simulink model "TorqueVectoring"  (R2020b)
settings: Solver=FixedStepAuto  StartTime=0.0  StopTime=Ts  FixedStep=0.001  RelTol=1e-3
PreLoadFcn:
  | setUpPurePursuitCurveHighVel
model workspace (MAT data in the model file):
  firstWarning = 0
  originalScenarioChecksum = 'F73A6DA3C723D3CA73A6F931B7A52A9C'
values from neighbouring files (symbols this model uses):
  Cf = 34282    [matlab.mat]    (also in matlab2.mat)
  Cr = 34282    [matlab.mat]    (also in matlab2.mat)
  g = 9.81    [matlab.mat]    (also in matlab2.mat)
  i = 5.45    [matlab.mat]    (also in matlab2.mat)
  Iz = 162    [matlab.mat]    (also in matlab2.mat)
  lf = 0.686    [matlab.mat]    (also in matlab2.mat)
  lr = 0.838    [matlab.mat]    (also in matlab2.mat)
  m = 300    [matlab.mat]    (also in matlab2.mat)
  period = 0.01    [matlab2.mat]
  Rw = 0.265    [matlab.mat]    (also in matlab2.mat)
  sigma = 1    [matlab.mat]    (also in matlab2.mat)
  tr = 0.549    [matlab.mat]    (also in matlab2.mat)
undefined symbols (not defined in the file or in its folder): Kd, Ki, Kp, MMax
libraries: simulink x2, vehdynlibsteering x1, pid_lib x1
settings Model: EnablePacing=on  PacingRate=0.450000  Creator=valakshe  LastModifiedBy=lugh8
settings SolverCC: ZeroCrossAlgorithm=Adaptive  PositivePriorityOrder=on
settings DataIOCC: SaveOutput=off  SaveTime=off
settings OptimizationCC: DefaultParameterBehavior=Inlined  UseDivisionForNetSlopeComputation=on  GainParamInheritBuiltInType=on  UseFloatMulNetSlope=on  InlineInvariantSignals=on  PassReuseOutputArgsAs=Individual arguments  ZeroExternalMemoryAtStartup=off  ZeroInternalMemoryAtStartup=off  NoFixptDivByZeroProtection=on  EfficientFloat2IntCast=on  LifeSpan=1  MaxStackSize=64  OptimizeBlockOrder=speed  DifferentSizesBufferReuse=on  EfficientTunableParamExpr=on
settings DebuggingCC: IgnoredZcDiagnostic=none  ParameterTunabilityLossMsg=error
settings HardwareCC: ProdBitPerPointer=32  ProdBitPerSizeT=32  ProdBitPerPtrDiffT=32  ProdLargestAtomicInteger=Long  ProdLargestAtomicFloat=Double  ProdWordSize=32  ProdLongLongMode=on  ProdHWDeviceType=ARM Compatible->ARM Cortex-M  HardwareBoardFeatureSet=SoCBlockset
settings SFSimCC: MATLABDynamicMemAlloc=off
settings RTWCC: Description=Embedded Coder  SystemTargetFile=ert.tlc  GenCodeOnly=on  PackageGeneratedCodeAndArtifacts=on  TemplateMakefile=ert_default_tmf
settings CodeAppCC: ForceParamTrailComments=on  IgnoreCustomStorageClasses=off  OperatorAnnotations=on  SimulinkDataObjDesc=on  SFDataObjDesc=on  CustomSymbolStrGlobalVar=rt$N$M  CustomSymbolStrType=$N$M  CustomSymbolStrFcn=$N$M$F  CustomSymbolStrMacro=$N$M  InsertBlockDesc=on
settings ERTTargetCC: IncludeMdlTerminateFcn=off  CombineSignalStateStructs=on  SupportAbsoluteTime=off  SupportComplex=off  SupportContinuousTime=on  SupportNonInlinedSFcns=on  InlinedParameterPlacement=NonHierarchical  ERTCustomFileTemplate=example_file_process.tlc  ERTFilePackagingFormat=CompactWithDataFile

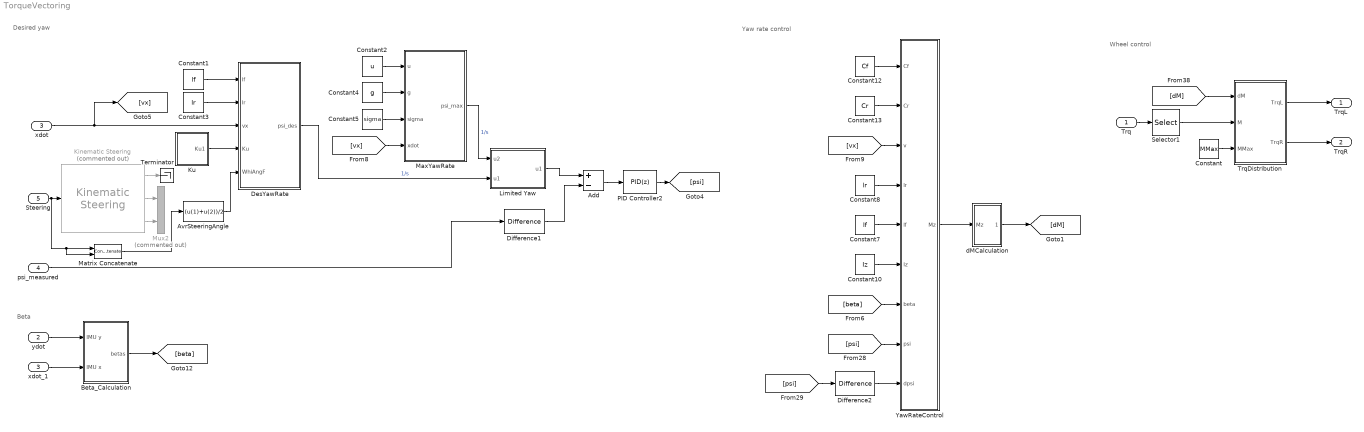
== system TorqueVectoring ==
  note: Desired yaw
  note: Beta
  note: Yaw rate control
  note: Wheel control
  Trq : Inport  OutDataTypeStr=double  PortDimensions=4  SampleTime=0
  ydot : Inport  Port=2  OutDataTypeStr=double  PortDimensions=1  SampleTime=0
  xdot : Inport  Port=3  OutDataTypeStr=double  PortDimensions=1  SampleTime=0
  psi_measured : Inport  Port=4  OutDataTypeStr=double  PortDimensions=1
  Steering : Inport  Port=5  OutDataTypeStr=double  PortDimensions=[1 1]  SampleTime=0
  Add : Sum  Inputs=+-
  AvrSteeringAngle : Fcn  Expr=(u(1)+u(2))/2
  Beta_Calculation : Subsystem
  Constant : Constant  Value=MMax
  Constant1 : Constant  Value=lf
  Constant10 : Constant  Value=Iz
  Constant12 : Constant  Value=Cf
  Constant13 : Constant  Value=Cr
  Constant2 : Constant  Value=u
  Constant3 : Constant  Value=lr
  Constant4 : Constant  Value=g
  Constant5 : Constant  Value=sigma
  Constant7 : Constant  Value=lf
  Constant8 : Constant  Value=lr
  DesYawRate : MATLAB Function  TreatAsAtomicUnit=on
  Difference1 : simulink/Discrete/Difference  ICPrevInput=0.0  OutMin=[]  OutMax=[]  OutDataType=fixdt(1, 16)  OutScaling=2^-10  DoSatur=off
  Difference2 : simulink/Discrete/Difference  ICPrevInput=0.0  OutMin=[]  OutMax=[]  OutDataType=fixdt(1, 16)  OutScaling=2^-10  DoSatur=off
  Kinematic Steering : vehdynlibsteering/Kinematic Steering  Commented=on  StrgType=Ackerman  StrgRatioType=Constant  Loc=Front  NrmlFctr=0.01  TrckWdth=1.098  WhlBase=L  Db=0  StrgRng=3.665  StrgAngBpts="[-6.2832   -5.0265   -3.7699   -2.5133   -1.2566         0    1.2566    2.5133    3.7699    5.0265    6.2832]"  StrgRatioTbl=|  StrgRatio=SR  StrgArmLngth=0.08  RckCsLngth=0.29  TieRodLngth=0.458  D=0.03  PnnRadius=0.019  PnnRadiusTbl="[0.0055    0.0055    0.0056    0.0057    0.0058    0.0057    0.0057    0.0057    0.0056    0.0055    0.0055]"  RodLngth=0.1  ParaArmLngth=0.9  aMode=2
      | [13.5000   13.3750   13.2500   13.1250   13.0000   13.0000   13.0000   13.1250   13.2500   13.3750   13.5000
      | ]
  Ku : Subsystem
  Limited Yaw : MATLAB Function  TreatAsAtomicUnit=on
  Matrix Concatenate : Concatenate
  MaxYawRate : MATLAB Function  TreatAsAtomicUnit=on
  Mux2 : Mux  Commented=on  Inputs=2
  PID Controller2 : pid_lib/PID Controller  Controller=PID  Form=Parallel  TimeDomain=Discrete-time  UseExternalTs=off  SampleTime=period  IntegratorMethod=Forward Euler  FilterMethod=Forward Euler  ControllerParametersSource=internal  P=Kp  I=Ki  D=Kd  UseFilter=on  N=10  TunerSelectOption=Transfer Function Based (PID Tuner App)  InitialConditionSource=internal  InitialConditionForIntegrator=0  InitialConditionForFilter=0  DifferentiatorICPrevScaledInput=0  ExternalReset=none  TrackingMode=off  Kt=1  LimitOutput=on  SatLimitsSource=internal  UpperSaturationLimit=inf  LowerSaturationLimit=-inf  LinearizeAsGain=on  AntiWindupMode=clamping  Kb=1  POutMin=[]  POutMax=[]  IOutMin=[]  IOutMax=[]  DOutMin=[]  DOutMax=[]  NOutMin=[]  NOutMax=[]  SumOutMin=[]  SumOutMax=[]  SaturationOutMin=[]  SaturationOutMax=[]  PParamMin=[]  PParamMax=[]  IParamMin=[]  IParamMax=[]  DParamMin=[]  DParamMax=[]  NParamMin=[]  NParamMax=[]  KbParamMin=[]  KbParamMax=[]  KtParamMin=[]  KtParamMax=[]  KbOutMin=[]  KbOutMax=[]  KtOutMin=[]  KtOutMax=[]  IntegratorOutMin=[]  IntegratorOutMax=[]  FilterOutMin=[]  FilterOutMax=[]  SumI1OutMin=[]  SumI1OutMax=[]  SumI2OutMin=[]  SumI2OutMax=[]  SumI3OutMin=[]  SumI3OutMax=[]  SumI4OutMin=[]  SumI4OutMax=[]  SumDOutMin=[]  SumDOutMax=[]  DifferentiatorOutMin=[]  DifferentiatorOutMax=[]  FilterDiffOutCoefMin=[]  FilterDiffOutCoefMax=[]  ReciprocalOutMin=[]  ReciprocalOutMax=[]  SumDenOutMin=[]  SumDenOutMax=[]  SumNumOutMin=[]  SumNumOutMax=[]  DivideOutMin=[]  DivideOutMax=[]  UdiffTsProdOutMin=[]  UdiffTsProdOutMax=[]  NTsProdOutMin=[]  NTsProdOutMax=[]  UintegralTsProdOutMin=[]  UintegralTsProdOutMax=[]  UngainTsProdOutMin=[]  UngainTsProdOutMax=[]  IntegratorContinuousStateAttributes=''  IntegratorStateMustResolveToSignalObject=off  IntegratorRTWStateStorageClass=Auto  FilterContinuousStateAttributes=''  FilterStateMustResolveToSignalObject=off  FilterRTWStateStorageClass=Auto  ParallelPVariant=InternalParameters  IdealPVariant=Disabled  IVariant=InternalParameters  DVariant=InternalParameters  IntegratorVariant=Discrete  SatVariant=Enabled  AWVariant=DiscClampingParallel  PCopyVariant=Disabled  TRVariant=Disabled  FdbkBlocksVariant=Forward  IdealPFdbkVariant=Disabled  SatFdbkVariant=Disabled  DerivativeFilterVariant=ForwardEulerFilter  NVariant=InternalParameters  NCopyVariant=Disabled  FilterICVariant=InternalICsFilter  IntegratorICVariant=InternalICs  ExternalResetVariant=Disabled  TRSumVariant=Passthrough  SumFdbkVariant=Disabled  SumVariant=Sum_PID  TsampFilterVariant=InternalTs  TsampNgainVariant=Passthrough  TsampIntegralVariant=Passthrough  ExternalSaturationOutDataTypeStr=Inherit: Same as second input
  Selector1 : Selector  InputPortWidth=4  IndexOptions=Index vector (dialog)  Indices=[3]  OutputSizes=1
  Terminator : Terminator
  TrqDistribution : MATLAB Function  TreatAsAtomicUnit=on
  YawRateControl : MATLAB Function  TreatAsAtomicUnit=on
  dMCalculation : Subsystem
  xdot_1 : InportShadow  Port=3  OutDataTypeStr=double  PortDimensions=1  SampleTime=0
  TrqL : Outport
  TrqR : Outport  Port=2
  wires:
  [psi] -> YawRateControl/8(psi)
  Constant12/1 -> YawRateControl/1(Cf)
  Trq/1 -> Selector1/1
  xdot/1 -> DesYawRate/3(vx), [vx]
  Constant3/1 -> DesYawRate/2(lr)
  psi_measured/1 -> Difference1/1
  Constant4/1 -> MaxYawRate/2(g)
  DesYawRate/1(psi_des) -> Limited Yaw/2("u1 ")  "1/s"
  [vx] -> YawRateControl/3(v)
  Constant2/1 -> MaxYawRate/1(u)
  YawRateControl/1(Mz) -> dMCalculation/1(Mz)
  Constant5/1 -> MaxYawRate/3(sigma)
  [psi] -> Difference2/1
  [dM] -> TrqDistribution/1(dM)
  Constant13/1 -> YawRateControl/2(Cr)
  Constant8/1 -> YawRateControl/4(lr)
  Constant7/1 -> YawRateControl/5(lf)
  Constant1/1 -> DesYawRate/1(lf)
  AvrSteeringAngle/1 -> DesYawRate/5(WhiAngF)
  MaxYawRate/1(psi_max) -> Limited Yaw/1(u2)  "1/s"
  [beta] -> YawRateControl/7(beta)
  Ku/1(Ku1) -> DesYawRate/4(Ku)
  ydot/1 -> Beta_Calculation/1(IMU y)
  Constant10/1 -> YawRateControl/6(Iz)
  xdot_1/1 -> Beta_Calculation/2(IMU x)
  Selector1/1 -> TrqDistribution/2(M)
  [vx] -> MaxYawRate/4(xdot)
  Difference2/1 -> YawRateControl/9(dpsi)
  TrqDistribution/1(TrqL) -> TrqL/1
  TrqDistribution/2(TrqR) -> TrqR/1
  PID Controller2/1 -> [psi]
  dMCalculation/1(dM1) -> [dM]
  Limited Yaw/1(u1) -> Add/1
  Difference1/1 -> Add/2
  Add/1 -> PID Controller2/1
  Beta_Calculation/1(betas) -> [beta]
  Constant/1 -> TrqDistribution/3(MMax)
  Steering/1 -> Matrix Concatenate/2, Matrix Concatenate/1, Kinematic Steering/1
  Kinematic Steering/3 -> Mux2/2
  Kinematic Steering/2 -> Mux2/1
  Kinematic Steering/1 -> Terminator/1
  Matrix Concatenate/1 -> AvrSteeringAngle/1

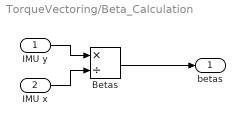
== system TorqueVectoring/Beta_Calculation ==
  IMU y : Inport
  IMU x : Inport  Port=2
  Betas : Product  Inputs=*/
  betas : Outport
  wires:
  Betas/1 -> betas/1
  IMU x/1 -> Betas/2
  IMU y/1 -> Betas/1

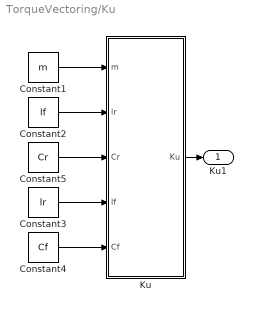
== system TorqueVectoring/Ku ==
  Constant1 : Constant  Value=m
  Constant2 : Constant  Value=lf
  Constant3 : Constant  Value=lr
  Constant4 : Constant  Value=Cf
  Constant5 : Constant  Value=Cr
  Ku : MATLAB Function  TreatAsAtomicUnit=on
  Ku1 : Outport
  wires:
  Constant4/1 -> Ku/5(Cf)
  Constant1/1 -> Ku/1(m)
  Constant3/1 -> Ku/4(lf)
  Constant2/1 -> Ku/2(lr)
  Constant5/1 -> Ku/3(Cr)
  Ku/1(Ku) -> Ku1/1

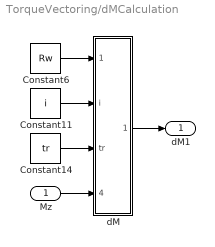
== system TorqueVectoring/dMCalculation ==
  Mz : Inport
  Constant11 : Constant  Value=i
  Constant14 : Constant  Value=tr
  Constant6 : Constant  Value=Rw
  dM : MATLAB Function  TreatAsAtomicUnit=on
  dM1 : Outport
  wires:
  Constant11/1 -> dM/2(i)
  Mz/1 -> dM/4(Mz)
  Constant6/1 -> dM/1(Rw)
  Constant14/1 -> dM/3(tr)
  dM/1(dM) -> dM1/1

== matlab function TorqueVectoring/Limited Yaw ==
  data: u2 input; u1 input; u1 output
function u1 = fcn(u2, u1)
%#codegen

if u1>=0
   u1 = min (u1, u2) ;  
   
else
    u1 = max (u1, -u2) ;
end

== matlab function TorqueVectoring/Ku/Ku ==
  data: m input; Ku output; lr input; Cr input; lf input; Cf input
function Ku = fcn(m, lr, Cr, lf, Cf)
%#codegen

Ku = (lr*m)/((lf+lr)^2 *Cf)-(lf*m)/((lf+lr)^2 *Cr);

== matlab function TorqueVectoring/YawRateControl ==
  data: Cf input; Mz output; Cr input; v input; lr input; lf input; Iz input; beta input; psi input; dpsi input
function Mz = fcn(Cf, Cr, v, lr, lf, Iz, beta, psi, dpsi)

Mz = Iz * dpsi + (Cf*lf - Cr*lr)* beta + 1/v*(lf^2*Cf + lr^2*Cr)*psi;

== matlab function TorqueVectoring/MaxYawRate ==
  data: u input; psi_max output; g input; sigma input; xdot input
function psi_max = fcn(u, g, sigma, xdot)
%#codegen

if xdot<= 0
    psi_max = 0;
else 
    psi_max = sigma * g * u / xdot;
end

== matlab function TorqueVectoring/DesYawRate ==
  data: lf input; psi_des output; lr input; vx input; Ku input; WhiAngF input
function psi_des = fcn( lf, lr , vx, Ku, WhiAngF)
%#codegen


psi_des = vx/((lf + lr) + Ku * vx^2) * WhiAngF;

== matlab function TorqueVectoring/dMCalculation/dM ==
  data: Rw input; dM output; i input; tr input; Mz input
function dM = fcn( Rw, i, tr, Mz)
%#codegen

dM = Mz * Rw / (2 * i * tr);

== matlab function TorqueVectoring/TrqDistribution ==
  data: dM input; M input; TrqL output; TrqR output; MMax input
function [TrqL,TrqR] = fcn(dM,M,MMax)
%#codegen

if M<=0 
   TrqL = 0;
   TrqR = 0;
else
    if dM>=0
        TrqL = M + dM/2;
        TrqR = M - dM/2;
    else
        TrqL = M + dM/2;
        TrqR = M - dM/2;
    end
end
if TrqL+TrqR >= MMax
    delta = (TrqL + TrqR)/2 - MMax/2;
    TrqL = TrqL - delta;
    TrqR = TrqR - delta;
else
end
